simulink model "p_inv_sub_coupled"  (Simulink 9.0)
settings: Solver=ode45  StartTime=0.0  StopTime=300  FixedStep=0.0001  MaxStep=0.001  RelTol=1e-6  AbsTol=1e-6
settings Model: Creator=Erick  LastModifiedBy=Erick
settings DataIOCC: SaveFormat=Dataset
settings OptimizationCC: LifeSpan=auto
settings DebuggingCC: UnderspecifiedInitializationDetection=Simplified  MergeDetectMultiDrivingBlocksExec=error  SFUnexpectedBacktrackingDiag=error  SFNoUnconditionalDefaultTransitionDiag=error  SFExecutionAtInitializationDiag=warning
settings HardwareCC: ProdBitPerPointer=64  ProdBitPerSizeT=64  ProdBitPerPtrDiffT=64  ProdLargestAtomicFloat=Float  ProdIntDivRoundTo=Zero  ProdEndianess=LittleEndian  ProdWordSize=64  ProdHWDeviceType=Intel->x86-64 (Windows64)
settings ModelReferenceCC: PropagateSignalLabelsOutOfModel=on
settings CodeAppCC: StateflowObjectComments=off
settings GRTTargetCC: TargetLangStandard=C99 (ISO)
settings ConfigComp: CovMetricSettings=dwe  CovHtmlReporting=off  CovSaveCumulativeToWorkspaceVar=off  CovSaveSingleToWorkspaceVar=off  CovExternalEMLEnable=on

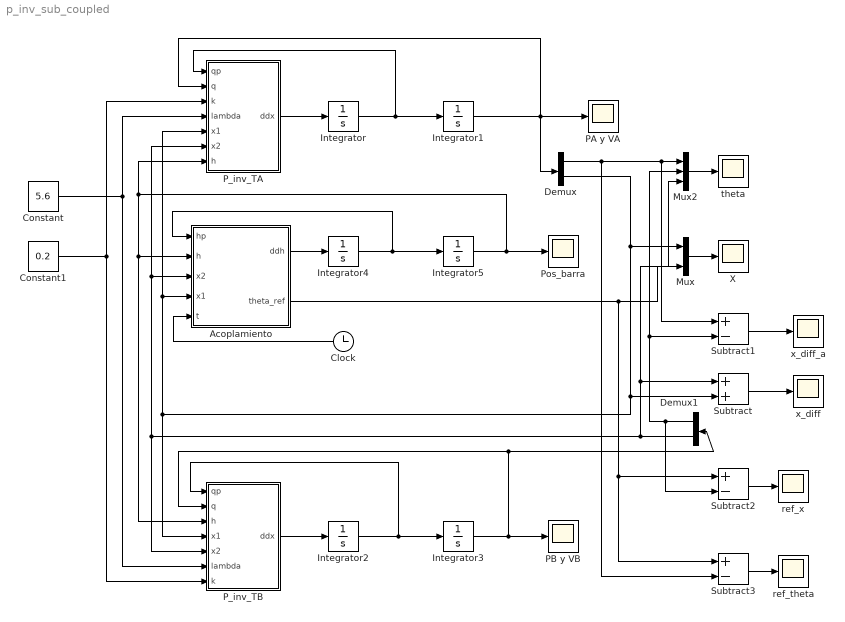
== system p_inv_sub_coupled ==
  Acoplamiento : MATLAB Function  TreatAsAtomicUnit=on
  Clock : Clock
  Constant : Constant  Value=5.6
  Constant1 : Constant  Value=0.2
  Demux : Demux  Outputs=2
  Demux1 : Demux  Outputs=2
  Integrator : Integrator  InitialCondition=[0 0]
  Integrator1 : Integrator  InitialCondition="[-0.1  0]"
  Integrator2 : Integrator  InitialCondition=[0 0]
  Integrator3 : Integrator  InitialCondition="[0.04  0]"
  Integrator4 : Integrator
  Integrator5 : Integrator
  Mux : Mux  Inputs=2
  Mux2 : Mux  Inputs=3
  PA y VA : Scope
  PB y VB : Scope
  P_inv_TA : MATLAB Function  TreatAsAtomicUnit=on
  P_inv_TB : MATLAB Function  TreatAsAtomicUnit=on
  Pos_barra : Scope
  Subtract : Sum
  Subtract1 : Sum  Inputs=+-
  Subtract2 : Sum  Inputs=+-
  Subtract3 : Sum  Inputs=+-
  X : Scope
  ref_theta : Scope
  ref_x : Scope
  theta : Scope
  x_diff : Scope
  x_diff_a : Scope
  wires:
  P_inv_TA/1(ddx) -> Integrator/1
  Integrator1/1 -> P_inv_TA/2(q), PA y VA/1, Demux/1
  Integrator/1 -> Integrator1/1, P_inv_TA/1(qp)
  Integrator2/1 -> P_inv_TB/1(qp), Integrator3/1
  P_inv_TB/1(ddx) -> Integrator2/1
  Integrator3/1 -> PB y VB/1, Demux1/1, P_inv_TB/2(q)
  Integrator4/1 -> Acoplamiento/1(hp), Integrator5/1
  Acoplamiento/1(ddh) -> Integrator4/1
  Mux/1 -> X/1
  Demux/2 -> Subtract/2, Acoplamiento/4(x1), P_inv_TA/5(x1), P_inv_TB/4(x1), Mux/1
  Demux1/2 -> Mux/2, Subtract/1, Acoplamiento/3(x2), P_inv_TA/6(x2), P_inv_TB/5(x2)
  Clock/1 -> Acoplamiento/5(t)
  Acoplamiento/2(theta_ref) -> Mux2/3, Subtract2/1, Subtract3/1
  Integrator5/1 -> Pos_barra/1, P_inv_TB/3(h), Acoplamiento/2(h), P_inv_TA/7(h)
  Mux2/1 -> theta/1
  Demux/1 -> Subtract1/1, Mux2/1, Subtract3/2
  Constant1/1 -> P_inv_TB/7(k), P_inv_TA/3(k)
  Constant/1 -> P_inv_TB/6(lambda), P_inv_TA/4(lambda)
  Subtract/1 -> x_diff/1
  Subtract1/1 -> x_diff_a/1
  Demux1/1 -> Subtract2/2, Mux2/2, Subtract1/2
  Subtract3/1 -> ref_theta/1
  Subtract2/1 -> ref_x/1

== matlab function P_inv_TB ==
  data: qp input double; q input double; ddx output double; h input double; x1 input double; x2 input double; lambda input double; k input double
function ddx = fcn(qp,q,h,x1,x2,lambda,k)
% function ddx = fcn(qp,q,h,x1,x2)

theta = q(1);
x = q(2);
thetap = qp(1);
xp = qp(2);

% parametros
g = 9.81;       % m/s^2
m1 = 1.785;     % kg
m2 = 0.213;     % kg
l1 = 0.330;     % m
lc1 = -0.0376;  % m
I1I2 = 0.0246;  % kgm^2

% parametros para resultados experimentales
% % k1 = 16.07;
% % k2 = 46.52;
% % k3 = 4.29;
% % k4 = 9.58;
% % lambda = 0;     % max 7.2 o falla
% % gamma = 0.25;

% parámetros para resultados numericos
k1 = 2.2409;
k2 = 2.1235;
% k1 = 0.7996;
% k2 = 0.7996;
k3 = 0.1854;
k4 = 1.5353;

% lambda =  5.5;   
gamma = 0.2025;
% gamma = 0.1163;
sigma = 0; % -5:fase; 5:anti-fase
% sigma = 20;
% k = 0.251;


% Señal de control
u = -k1*theta-k2*x-k3*thetap-k4*xp-lambda*(x^2+xp^2-gamma)*xp+sigma*h+k*(x2+x1);
% u = 0;

M = [I1I2+(x^2+l1^2)*m2-m1*lc1^2 l1*m2;
     l1*m2 m2]; % Matriz de inercia

C = [2*m2*x*xp 0;
    -m2*thetap*x 0]*[thetap;xp]; % Matriz de coriolis

G=[-m2*g*cos(theta)*x-(l1*m2+m1*lc1)*g*sin(theta);
    -m2*g*sin(theta)]; % Matriz de fuerzas gravitacionales

tau = [0; u]; % torque de control (sub actuado)
   
% Fric_viscosa = 0.01*qp; % no esta en el modelo, es para probar

F = tau-C-G; 
% F = tau+C*[thetap;xp]+G+Fric_viscosa; 

ddx = inv(M)*F;

== matlab function P_inv_TA ==
  data: qp input double; q input double; k input double; lambda input double; x1 input double; x2 input double; ddx output double; h input double
function ddx = fcn(qp,q,k,lambda,x1,x2,h)
% function ddx = fcn(qp,q,x1,x2,h)

theta = q(1);
x = q(2);
thetap = qp(1);
xp = qp(2);

% parametros
g = 9.81;       % m/s^2
m1 = 1.785;     % kg
m2 = 0.213;     % kg
l1 = 0.330;     % m
lc1 = -0.0376;  % m
I1I2 = 0.0246;  % kgm^2


% parametros para resultados experimentales
% % k1 = 16.07;
% % k2 = 46.52;
% % k3 = 4.29;
% % k4 = 9.58;
% % lambda = 0;     % max 7.2 o falla
% % gamma = 0.25;


% parámetros para resultados numericos
k1 = 2.2409;
k2 = 2.1235;
% k1 = 0.7996;
% k2 = 0.7996;
k3 = 0.1854;
k4 = 1.5353;


% lambda =  5.5;  % ?   
gamma = 0.2025;
% gamma = 0.1163;
sigma = 0; % -5:fase; 5:anti-fase
% sigma = 20;
% k = 0.251;


% Señal de control
u = -k1*theta-k2*x-k3*thetap-k4*xp-lambda*(x^2+xp^2-gamma)*xp+sigma*h+k*(x1+x2);


M = [I1I2+(x^2+l1^2)*m2-m1*lc1^2 l1*m2;
     l1*m2 m2]; % Matriz de inercia

C = [2*m2*x*xp 0;
    -m2*thetap*x 0]*[thetap;xp]; % Matriz de coriolis

G=[-m2*g*cos(theta)*x-(l1*m2+m1*lc1)*g*sin(theta);
    -m2*g*sin(theta)]; % Matriz de fuerzas gravitacionales

tau = [0;u]; % torque de control (sub actuado)
   
% Fric_viscosa = 0.01*qp; % no esta en el modelo, es para probar

F = tau-C-G; 
% F = tau+C*[thetap;xp]+G+Fric_viscosa; 

ddx = inv(M)*F;

== matlab function Acoplamiento ==
  data: hp input double; h input double; x2 input double; ddh output double; x1 input double; t input double; theta_ref output double
function [ddh,theta_ref] = fcn(hp,h,x2,x1,t)

% parametros
h1=45;  % r1
h2=3.1; % r2
% h1 = 0.4094;
% h2 = 0.4094;
mu=.35; % ?


% eta = 0.06; % ?
% w = 5.4611; % ?
% w = 6.2;


g = 9.81;       % m/s^2
m1 = 1.785;     % kg
m2 = 0.213;     % kg
l1 = 0.330;     % m
lc1 = -0.0376;  % m
I1I2 = 0.0246;  % kgm^2


% w = 6.6887;
% w = 6.0357;
% w = 6.0415;
w = 6.0357;
% eta = 0.0164142;
% eta = 0.024496;
eta = 0.034456;
theta_ref = eta*sin(w*t);


% theta_refp = eta*w*cos(w*t);
% theta_refpp = -eta*w^2*sin(w*t);

% F = 2*m1*lc1*(theta_refpp*cos(theta_ref)-theta_refp^2*sin(theta_ref));

ddh=-h1*h-h2*hp+mu*(x1+x2+2*theta_ref);
